simulink model "automatic_reset_counter"  (R2019b)
settings: Solver=VariableStepDiscrete  StartTime=0.0  StopTime=10.0  MaxStep=0.02  RelTol=1e-3
settings Model: Creator=Yinglongli  LastModifiedBy=Yinglongli

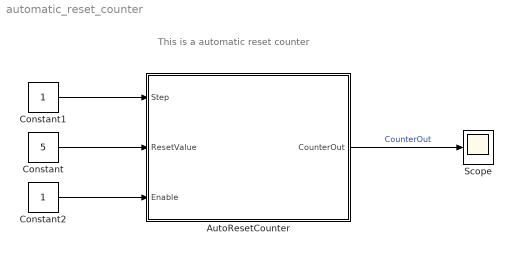
== system automatic_reset_counter ==
  note: This is a automatic reset counter
  AutoResetCounter : Subsystem
  Constant : Constant  Value=5
  Constant1 : Constant
  Constant2 : Constant
  Scope : Scope
  wires:
  Constant1/1 -> AutoResetCounter/1(Step)
  AutoResetCounter/1(CounterOut) -> Scope/1  "CounterOut"
  Constant/1 -> AutoResetCounter/2(ResetValue)
  Constant2/1 -> AutoResetCounter/3(Enable)

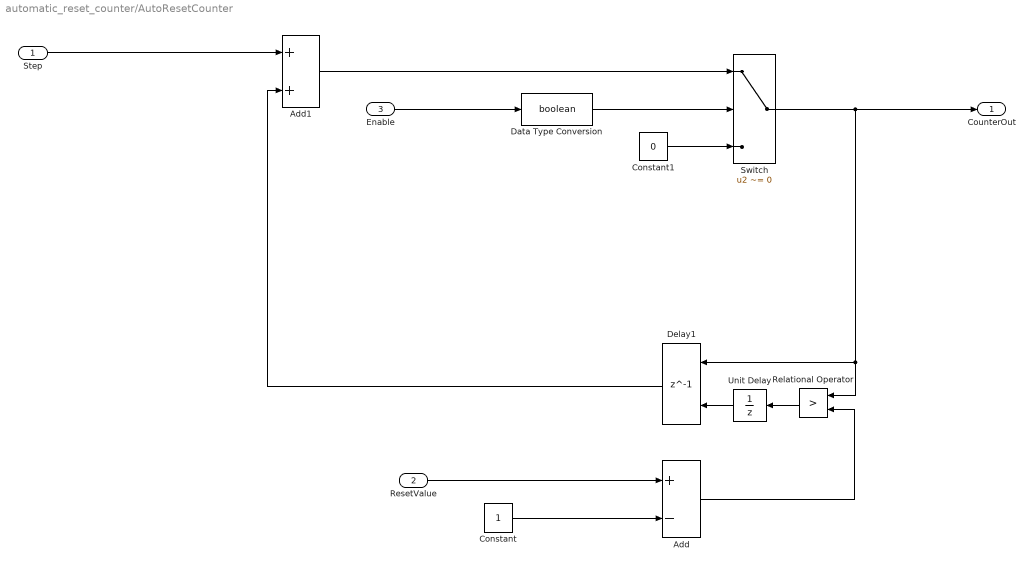
== system automatic_reset_counter/AutoResetCounter ==
  Step : Inport
  ResetValue : Inport  Port=2
  Enable : Inport  Port=3
  Add : Sum  Inputs=+-
  Add1 : Sum
  Constant : Constant
  Constant1 : Constant  Value=0
  Data Type Conversion : DataTypeConversion  OutDataTypeStr=boolean
  Delay1 : Delay  DelayLength=1  InitialCondition=0  ExternalReset=Rising
      settings: InputPortMap=u0,r5
  Relational Operator : RelationalOperator  Operator=>  OutDataTypeStr=boolean  RndMeth=Simplest
  Switch : Switch  Criteria=u2 ~= 0
  Unit Delay : UnitDelay  SampleTime=-1  HasFrameUpgradeWarning=on
  CounterOut : Outport
  wires:
  Unit Delay/1 -> Delay1/2
  Switch/1 -> Relational Operator/1, Delay1/1, CounterOut/1
  Delay1/1 -> Add1/2
  Relational Operator/1 -> Unit Delay/1
  Step/1 -> Add1/1
  ResetValue/1 -> Add/1
  Add/1 -> Relational Operator/2
  Constant/1 -> Add/2
  Enable/1 -> Data Type Conversion/1
  Data Type Conversion/1 -> Switch/2
  Add1/1 -> Switch/1
  Constant1/1 -> Switch/3
